simulink model "FSAC2021_V1_Running"  (R2014a)
settings: Solver=FixedStepDiscrete  StartTime=0.0  StopTime=inf  FixedStep=0.0005  RelTol=1e-3
model workspace (MAT data in the model file):
  MCOS : class17 (value not decoded)
  MCOS : class17 (value not decoded)
  MCOS : class17 (value not decoded)
  MCOS : class17 (value not decoded)
  MCOS : class17 (value not decoded)
  MCOS : class17 (value not decoded)
  MCOS : class17 (value not decoded)
  MCOS : class17 (value not decoded)
  MCOS : class17 (value not decoded)
  MCOS : class17 (value not decoded)
  MCOS : class17 (value not decoded)
  MCOS : class17 (value not decoded)
  MCOS : class17 (value not decoded)
  MCOS : class17 (value not decoded)
  MCOS : class17 (value not decoded)
  MCOS : class17 (value not decoded)
  MCOS : class17 (value not decoded)
  MCOS : class17 (value not decoded)
  MCOS : class17 (value not decoded)
  BUZZER_START = 1
  MCOS : class17 (value not decoded)
  MCOS : class17 (value not decoded)
  MCOS : class17 (value not decoded)
  MCOS : class17 (value not decoded)
  MCOS : class17 (value not decoded)
  MCOS : class17 (value not decoded)
  MCOS : class17 (value not decoded)
  MCOS : class17 (value not decoded)
  MCOS : class17 (value not decoded)
  MCOS : class17 (value not decoded)
  MCOS : class17 (value not decoded)
  MCOS : class17 (value not decoded)
  MCOS : class17 (value not decoded)
  MCOS : class17 (value not decoded)
  MCOS : class17 (value not decoded)
  MCOS : class17 (value not decoded)
  MCOS : class17 (value not decoded)
  MCOS : class17 (value not decoded)
  MCOS : class17 (value not decoded)
  MCOS : class17 (value not decoded)
  MCOS : class17 (value not decoded)
  MCOS : class17 (value not decoded)
  MCOS : class17 (value not decoded)
  MCOS : class17 (value not decoded)
  MCOS : class17 (value not decoded)
  MCOS : class17 (value not decoded)
  MCOS : class17 (value not decoded)
  MCOS : class17 (value not decoded)
  MCOS : class17 (value not decoded)
  MCOS : class17 (value not decoded)
  MCOS : class17 (value not decoded)
  MCOS : class17 (value not decoded)
  MCOS : class17 (value not decoded)
  MCOS : class17 (value not decoded)
  MCOS : class17 (value not decoded)
  MCOS : class17 (value not decoded)
  MCOS : class17 (value not decoded)
  MCOS : class17 (value not decoded)
  Brake = 11
  MCOS : class17 (value not decoded)
  MCOS : class17 (value not decoded)
  MCOS : class17 (value not decoded)
  MCOS : class17 (value not decoded)
  MCOS : class17 (value not decoded)
  MCOS : class17 (value not decoded)
  MCOS : class17 (value not decoded)
  MCOS : class17 (value not decoded)
  Sensor_Acc_b = 101.85
  Sensor_Acc_k = -0.0185
  Str_Sen_Orig_Angle = -341
  MCOS : class17 (value not decoded)
  Tire_D = 0.47
  T = 0.05
libraries: simulink x402, ec55xxlib x134
(part 3 of 17)

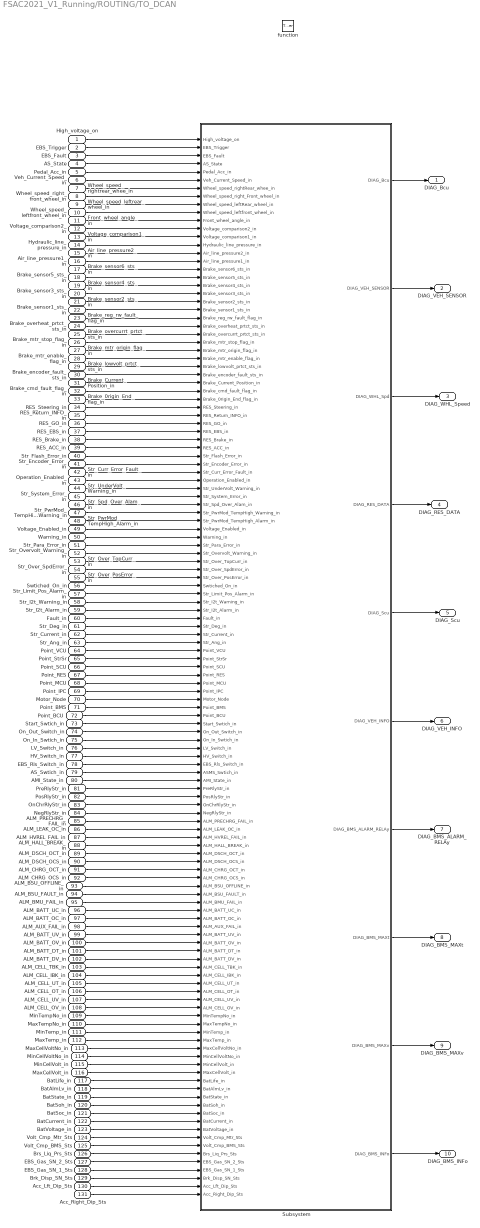
== system FSAC2021_V1_Running/ROUTING/TO_DCAN ==
  High_voltage_on : Inport
  EBS_Trigger : Inport  Port=2
  EBS_Fault : Inport  Port=3
  AS_State : Inport  Port=4
  Pedal_Acc_in : Inport  Port=5
  Veh_Current_Speed_in : Inport  Port=6
  Wheel_speed_rightrear_whee_in : Inport  Port=7
  Wheel_speed_right_front_wheel_in : Inport  Port=8
  Wheel_speed_leftrear_wheel_in : Inport  Port=9
  Wheel_speed_leftfront_wheel_in : Inport  Port=10
  Front_wheel_angle_in : Inport  Port=11
  Voltage_comparison2_in : Inport  Port=12
  Voltage_comparison1_in : Inport  Port=13
  Hydraulic_line_pressure_in : Inport  Port=14
  Air_line_pressure2_in : Inport  Port=15
  Air_line_pressure1_in : Inport  Port=16
  Brake_sensor6_sts_in : Inport  Port=17
  Brake_sensor5_sts_in : Inport  Port=18
  Brake_sensor4_sts_in : Inport  Port=19
  Brake_sensor3_sts_in : Inport  Port=20
  Brake_sensor2_sts_in : Inport  Port=21
  Brake_sensor1_sts_in : Inport  Port=22
  Brake_reg_rw_fault_flag_in : Inport  Port=23
  Brake_overheat_prtct_sts_in : Inport  Port=24
  Brake_overcurrt_prtct_sts_in : Inport  Port=25
  Brake_mtr_stop_flag_in : Inport  Port=26
  Brake_mtr_origin_flag_in : Inport  Port=27
  Brake_mtr_enable_flag_in : Inport  Port=28
  Brake_lowvolt_prtct_sts_in : Inport  Port=29
  Brake_encoder_fault_sts_in : Inport  Port=30
  Brake_Current_Position_in : Inport  Port=31
  Brake_cmd_fault_flag_in : Inport  Port=32
  Brake_0rigin_End_flag_in : Inport  Port=33
  RES_Steering_in : Inport  Port=34
  RES_Return_INFO_in : Inport  Port=35
  RES_GO_in : Inport  Port=36
  RES_EBS_in : Inport  Port=37
  RES_Brake_in : Inport  Port=38
  RES_ACC_in : Inport  Port=39
  Str_Flash_Error_in : Inport  Port=40
  Str_Encoder_Error_in : Inport  Port=41
  Str_Curr_Error_Fault_in : Inport  Port=42
  Operation_Enabled_in : Inport  Port=43
  Str_UnderVolt_Warning_in : Inport  Port=44
  Str_System_Error_in : Inport  Port=45
  Str_Spd_Over_Alam_in : Inport  Port=46
  Str_PwrMod_TempHigh_Warning_in : Inport  Port=47
  Str_PwrMod_TempHigh_Alarm_in : Inport  Port=48
  Voltage_Enabled_in : Inport  Port=49
  Warning_in : Inport  Port=50
  Str_Para_Error_in : Inport  Port=51
  Str_Overvolt_Warning_in : Inport  Port=52
  Str_Over_TopCurr_in : Inport  Port=53
  Str_Over_SpdError_in : Inport  Port=54
  Str_Over_PosError_in : Inport  Port=55
  Swtiched_On_in : Inport  Port=56
  Str_Limit_Pos_Alarm_in : Inport  Port=57
  Str_I2t_Warning_in : Inport  Port=58
  Str_I2t_Alarm_in : Inport  Port=59
  Fault_in : Inport  Port=60
  Str_Deg_in : Inport  Port=61
  Str_Current_in : Inport  Port=62
  Str_Ang_in : Inport  Port=63
  Point_VCU : Inport  Port=64
  Point_StrSr : Inport  Port=65
  Point_SCU : Inport  Port=66
  Point_RES : Inport  Port=67
  Point_MCU : Inport  Port=68
  Point_IPC : Inport  Port=69
  Motor_Node : Inport  Port=70
  Point_BMS : Inport  Port=71
  Point_BCU : Inport  Port=72
  Start_Swtich_in : Inport  Port=73
  On_Out_Switch_in : Inport  Port=74
  On_In_Swtich_in : Inport  Port=75
  LV_Switch_in : Inport  Port=76
  HV_Switch_in : Inport  Port=77
  EBS_Rls_Switch_in : Inport  Port=78
  AS_Swtich_in : Inport  Port=79
  AMI_State_in : Inport  Port=80
  PreRlyStr_in : Inport  Port=81
  PosRlyStr_in : Inport  Port=82
  OnChrRlyStr_in : Inport  Port=83
  NegRlyStr_in : Inport  Port=84
  ALM_PRECHRG_FAIL_in : Inport  Port=85
  ALM_LEAK_OC_in : Inport  Port=86
  ALM_HVREL_FAIL_in : Inport  Port=87
  ALM_HALL_BREAK_in : Inport  Port=88
  ALM_DSCH_OCT_in : Inport  Port=89
  ALM_DSCH_OCS_in : Inport  Port=90
  ALM_CHRG_OCT_in : Inport  Port=91
  ALM_CHRG_OCS_in : Inport  Port=92
  ALM_BSU_OFFLINE_in : Inport  Port=93
  ALM_BSU_FAULT_in : Inport  Port=94
  ALM_BMU_FAIL_in : Inport  Port=95
  ALM_BATT_UC_in : Inport  Port=96
  ALM_BATT_OC_in : Inport  Port=97
  ALM_AUX_FAIL_in : Inport  Port=98
  ALM_BATT_UV_in : Inport  Port=99
  ALM_BATT_OV_in : Inport  Port=100
  ALM_BATT_DT_in : Inport  Port=101
  ALM_BATT_DV_in : Inport  Port=102
  ALM_CELL_TBK_in : Inport  Port=103
  ALM_CELL_IBK_in : Inport  Port=104
  ALM_CELL_UT_in : Inport  Port=105
  ALM_CELL_OT_in : Inport  Port=106
  ALM_CELL_UV_in : Inport  Port=107
  ALM_CELL_OV_in : Inport  Port=108
  MinTempNo_in : Inport  Port=109
  MaxTempNo_in : Inport  Port=110
  MinTemp_in : Inport  Port=111
  MaxTemp_in : Inport  Port=112
  MaxCellVoltNo_in : Inport  Port=113
  MinCellVoltNo_in : Inport  Port=114
  MinCellVolt_in : Inport  Port=115
  MaxCellVolt_in : Inport  Port=116
  BatLife_in : Inport  Port=117
  BatAlmLv_in : Inport  Port=118
  BatState_in : Inport  Port=119
  BatSoh_in : Inport  Port=120
  BatSoc_in : Inport  Port=121
  BatCurrent_in : Inport  Port=122
  BatVoltage_in : Inport  Port=123
  Volt_Cmp_Mtr_Sts : Inport  Port=124
  Volt_Cmp_BMS_Sts : Inport  Port=125
  "Brs_Liq_Prs_Sts " : Inport  Port=126
  EBS_Gas_SN_2_Sts : Inport  Port=127
  EBS_Gas_SN_1_Sts : Inport  Port=128
  Brk_Disp_SN_Sts : Inport  Port=129
  Acc_Lft_Dip_Sts : Inport  Port=130
  Acc_Right_Dip_Sts : Inport  Port=131
  function : TriggerPort  TriggerType=function-call
  Subsystem : Subsystem
  DIAG_Bcu : Outport
  DIAG_VEH_SENSOR : Outport  Port=2
  DIAG_WHL_Speed : Outport  Port=3
  DIAG_RES_DATA : Outport  Port=4
  DIAG_Scu : Outport  Port=5
  DIAG_VEH_INFO : Outport  Port=6
  DIAG_BMS_ALARM_RELAy : Outport  Port=7
  DIAG_BMS_MAXt : Outport  Port=8
  DIAG_BMS_MAXv : Outport  Port=9
  DIAG_BMS_INFo : Outport  Port=10
  wires:
  High_voltage_on/1 -> Subsystem/1(High_voltage_on)
  EBS_Trigger/1 -> Subsystem/2(EBS_Trigger)
  EBS_Fault/1 -> Subsystem/3(EBS_Fault)
  AS_State/1 -> Subsystem/4(AS_State)
  Pedal_Acc_in/1 -> Subsystem/5(Pedal_Acc_in)
  Veh_Current_Speed_in/1 -> Subsystem/6(Veh_Current_Speed_in)
  Wheel_speed_rightrear_whee_in/1 -> Subsystem/7(Wheel_speed_rightRear_whee_in)
  Wheel_speed_right_front_wheel_in/1 -> Subsystem/8(Wheel_speed_right_Front_wheel_in)
  Wheel_speed_leftrear_wheel_in/1 -> Subsystem/9(Wheel_speed_leftRear_wheel_in)
  Wheel_speed_leftfront_wheel_in/1 -> Subsystem/10(Wheel_speed_leftfront_wheel_in)
  Front_wheel_angle_in/1 -> Subsystem/11(Front_wheel_angle_in)
  Voltage_comparison2_in/1 -> Subsystem/12(Voltage_comparison2_in)
  Voltage_comparison1_in/1 -> Subsystem/13(Voltage_comparison1_in)
  Hydraulic_line_pressure_in/1 -> Subsystem/14(Hydraulic_line_pressure_in)
  Air_line_pressure2_in/1 -> Subsystem/15(Air_line_pressure2_in)
  Air_line_pressure1_in/1 -> Subsystem/16(Air_line_pressure1_in)
  Brake_sensor6_sts_in/1 -> Subsystem/17(Brake_sensor6_sts_in)
  Brake_sensor5_sts_in/1 -> Subsystem/18(Brake_sensor5_sts_in)
  Brake_sensor4_sts_in/1 -> Subsystem/19(Brake_sensor4_sts_in)
  Brake_sensor3_sts_in/1 -> Subsystem/20(Brake_sensor3_sts_in)
  Brake_sensor2_sts_in/1 -> Subsystem/21(Brake_sensor2_sts_in)
  Brake_sensor1_sts_in/1 -> Subsystem/22(Brake_sensor1_sts_in)
  Brake_reg_rw_fault_flag_in/1 -> Subsystem/23(Brake_reg_rw_fault_flag_in)
  Brake_overheat_prtct_sts_in/1 -> Subsystem/24(Brake_overheat_prtct_sts_in)
  Brake_overcurrt_prtct_sts_in/1 -> Subsystem/25(Brake_overcurrt_prtct_sts_in)
  Brake_mtr_stop_flag_in/1 -> Subsystem/26(Brake_mtr_stop_flag_in)
  Brake_mtr_origin_flag_in/1 -> Subsystem/27(Brake_mtr_origin_flag_in)
  Brake_mtr_enable_flag_in/1 -> Subsystem/28(Brake_mtr_enable_flag_in)
  Brake_lowvolt_prtct_sts_in/1 -> Subsystem/29(Brake_lowvolt_prtct_sts_in)
  Brake_encoder_fault_sts_in/1 -> Subsystem/30(Brake_encoder_fault_sts_in)
  Brake_Current_Position_in/1 -> Subsystem/31(Brake_Current_Position_in)
  Brake_cmd_fault_flag_in/1 -> Subsystem/32(Brake_cmd_fault_flag_in)
  Brake_0rigin_End_flag_in/1 -> Subsystem/33(Brake_0rigin_End_flag_in)
  RES_Steering_in/1 -> Subsystem/34(RES_Steering_in)
  RES_Return_INFO_in/1 -> Subsystem/35(RES_Return_INFO_in)
  RES_GO_in/1 -> Subsystem/36(RES_GO_in)
  RES_EBS_in/1 -> Subsystem/37(RES_EBS_in)
  RES_Brake_in/1 -> Subsystem/38(RES_Brake_in)
  RES_ACC_in/1 -> Subsystem/39(RES_ACC_in)
  Str_Flash_Error_in/1 -> Subsystem/40(Str_Flash_Error_in)
  Str_Encoder_Error_in/1 -> Subsystem/41(Str_Encoder_Error_in)
  Str_Curr_Error_Fault_in/1 -> Subsystem/42(Str_Curr_Error_Fault_in)
  Operation_Enabled_in/1 -> Subsystem/43(Operation_Enabled_in)
  Str_UnderVolt_Warning_in/1 -> Subsystem/44(Str_UnderVolt_Warning_in)
  Str_System_Error_in/1 -> Subsystem/45(Str_System_Error_in)
  Str_Spd_Over_Alam_in/1 -> Subsystem/46(Str_Spd_Over_Alam_in)
  Str_PwrMod_TempHigh_Warning_in/1 -> Subsystem/47(Str_PwrMod_TempHigh_Warning_in)
  Str_PwrMod_TempHigh_Alarm_in/1 -> Subsystem/48(Str_PwrMod_TempHigh_Alarm_in)
  Voltage_Enabled_in/1 -> Subsystem/49(Voltage_Enabled_in)
  Warning_in/1 -> Subsystem/50(Warning_in)
  Str_Para_Error_in/1 -> Subsystem/51(Str_Para_Error_in)
  Str_Overvolt_Warning_in/1 -> Subsystem/52(Str_Overvolt_Warning_in)
  Str_Over_TopCurr_in/1 -> Subsystem/53(Str_Over_TopCurr_in)
  Str_Over_SpdError_in/1 -> Subsystem/54(Str_Over_SpdError_in)
  Str_Over_PosError_in/1 -> Subsystem/55(Str_Over_PosError_in)
  Swtiched_On_in/1 -> Subsystem/56(Swtiched_On_in)
  Str_Limit_Pos_Alarm_in/1 -> Subsystem/57(Str_Limit_Pos_Alarm_in)
  Str_I2t_Warning_in/1 -> Subsystem/58(Str_I2t_Warning_in)
  Str_I2t_Alarm_in/1 -> Subsystem/59(Str_I2t_Alarm_in)
  Fault_in/1 -> Subsystem/60(Fault_in)
  Str_Deg_in/1 -> Subsystem/61(Str_Deg_in)
  Str_Current_in/1 -> Subsystem/62(Str_Current_in)
  Str_Ang_in/1 -> Subsystem/63(Str_Ang_in)
  Point_VCU/1 -> Subsystem/64(Point_VCU)
  Point_StrSr/1 -> Subsystem/65(Point_StrSr)
  Point_SCU/1 -> Subsystem/66(Point_SCU)
  Point_RES/1 -> Subsystem/67(Point_RES)
  Point_MCU/1 -> Subsystem/68(Point_MCU)
  Point_IPC/1 -> Subsystem/69(Point_IPC)
  Point_BMS/1 -> Subsystem/71(Point_BMS)
  Point_BCU/1 -> Subsystem/72(Point_BCU)
  Start_Swtich_in/1 -> Subsystem/73(Start_Swtich_in)
  On_Out_Switch_in/1 -> Subsystem/74(On_Out_Switch_in)
  On_In_Swtich_in/1 -> Subsystem/75(On_In_Swtich_in)
  LV_Switch_in/1 -> Subsystem/76(LV_Switch_in)
  HV_Switch_in/1 -> Subsystem/77(HV_Switch_in)
  EBS_Rls_Switch_in/1 -> Subsystem/78(EBS_Rls_Switch_in)
  AS_Swtich_in/1 -> Subsystem/79(ASMS_Swtich_in)
  AMI_State_in/1 -> Subsystem/80(AMI_State_in)
  PreRlyStr_in/1 -> Subsystem/81(PreRlyStr_in)
  PosRlyStr_in/1 -> Subsystem/82(PosRlyStr_in)
  OnChrRlyStr_in/1 -> Subsystem/83(OnChrRlyStr_in)
  NegRlyStr_in/1 -> Subsystem/84(NegRlyStr_in)
  ALM_PRECHRG_FAIL_in/1 -> Subsystem/85(ALM_PRECHRG_FAIL_in)
  ALM_LEAK_OC_in/1 -> Subsystem/86(ALM_LEAK_OC_in)
  ALM_HVREL_FAIL_in/1 -> Subsystem/87(ALM_HVREL_FAIL_in)
  ALM_HALL_BREAK_in/1 -> Subsystem/88(ALM_HALL_BREAK_in)
  ALM_DSCH_OCT_in/1 -> Subsystem/89(ALM_DSCH_OCT_in)
  ALM_DSCH_OCS_in/1 -> Subsystem/90(ALM_DSCH_OCS_in)
  ALM_CHRG_OCT_in/1 -> Subsystem/91(ALM_CHRG_OCT_in)
  ALM_CHRG_OCS_in/1 -> Subsystem/92(ALM_CHRG_OCS_in)
  ALM_BSU_OFFLINE_in/1 -> Subsystem/93(ALM_BSU_OFFLINE_in)
  ALM_BSU_FAULT_in/1 -> Subsystem/94(ALM_BSU_FAULT_in)
  ALM_BMU_FAIL_in/1 -> Subsystem/95(ALM_BMU_FAIL_in)
  ALM_BATT_UC_in/1 -> Subsystem/96(ALM_BATT_UC_in)
  ALM_BATT_OC_in/1 -> Subsystem/97(ALM_BATT_OC_in)
  ALM_AUX_FAIL_in/1 -> Subsystem/98(ALM_AUX_FAIL_in)
  ALM_BATT_UV_in/1 -> Subsystem/99(ALM_BATT_UV_in)
  ALM_BATT_OV_in/1 -> Subsystem/100(ALM_BATT_OV_in)
  ALM_BATT_DT_in/1 -> Subsystem/101(ALM_BATT_DT_in)
  ALM_BATT_DV_in/1 -> Subsystem/102(ALM_BATT_DV_in)
  ALM_CELL_TBK_in/1 -> Subsystem/103(ALM_CELL_TBK_in)
  ALM_CELL_IBK_in/1 -> Subsystem/104(ALM_CELL_IBK_in)
  ALM_CELL_UT_in/1 -> Subsystem/105(ALM_CELL_UT_in)
  ALM_CELL_OT_in/1 -> Subsystem/106(ALM_CELL_OT_in)
  ALM_CELL_UV_in/1 -> Subsystem/107(ALM_CELL_UV_in)
  ALM_CELL_OV_in/1 -> Subsystem/108(ALM_CELL_OV_in)
  MinTempNo_in/1 -> Subsystem/109(MinTempNo_in)
  MaxTempNo_in/1 -> Subsystem/110(MaxTempNo_in)
  MinTemp_in/1 -> Subsystem/111(MinTemp_in)
  MaxTemp_in/1 -> Subsystem/112(MaxTemp_in)
  MaxCellVoltNo_in/1 -> Subsystem/113(MaxCellVoltNo_in)
  MinCellVoltNo_in/1 -> Subsystem/114(MinCellVoltNo_in)
  MinCellVolt_in/1 -> Subsystem/115(MinCellVolt_in)
  MaxCellVolt_in/1 -> Subsystem/116(MaxCellVolt_in)
  BatLife_in/1 -> Subsystem/117(BatLife_in)
  BatAlmLv_in/1 -> Subsystem/118(BatAlmLv_in)
  BatState_in/1 -> Subsystem/119(BatState_in)
  BatSoh_in/1 -> Subsystem/120(BatSoh_in)
  BatSoc_in/1 -> Subsystem/121(BatSoc_in)
  BatCurrent_in/1 -> Subsystem/122(BatCurrent_in)
  BatVoltage_in/1 -> Subsystem/123(BatVoltage_in)
  Subsystem/1(DIAG_Bcu) -> DIAG_Bcu/1
  Subsystem/2("DIAG_VEH_SENSOR ") -> DIAG_VEH_SENSOR/1
  Subsystem/3(DIAG_WHL_Spd) -> DIAG_WHL_Speed/1
  Subsystem/4(DIAG_RES_DATA) -> DIAG_RES_DATA/1
  Subsystem/5(DIAG_Scu) -> DIAG_Scu/1
  Subsystem/6("DIAG_VEH_INFO ") -> DIAG_VEH_INFO/1
  Subsystem/7(DIAG_BMS_ALARM_RELAy) -> DIAG_BMS_ALARM_RELAy/1
  Subsystem/8(DIAG_BMS_MAXt) -> DIAG_BMS_MAXt/1
  Subsystem/9(DIAG_BMS_MAXv) -> DIAG_BMS_MAXv/1
  Subsystem/10(DIAG_BMS_INFo) -> DIAG_BMS_INFo/1
  Motor_Node/1 -> Subsystem/70(Motor_Node)
  Volt_Cmp_Mtr_Sts/1 -> Subsystem/124(Volt_Cmp_Mtr_Sts)
  Volt_Cmp_BMS_Sts/1 -> Subsystem/125(Volt_Cmp_BMS_Sts)
  "Brs_Liq_Prs_Sts "/1 -> Subsystem/126("Brs_Liq_Prs_Sts ")
  EBS_Gas_SN_2_Sts/1 -> Subsystem/127(EBS_Gas_SN_2_Sts)
  EBS_Gas_SN_1_Sts/1 -> Subsystem/128(EBS_Gas_SN_1_Sts)
  Brk_Disp_SN_Sts/1 -> Subsystem/129(Brk_Disp_SN_Sts)
  Acc_Lft_Dip_Sts/1 -> Subsystem/130(Acc_Lft_Dip_Sts)
  Acc_Right_Dip_Sts/1 -> Subsystem/131(Acc_Right_Dip_Sts)

== system FSAC2021_V1_Running/ROUTING/TO_PCAN ==
  function : TriggerPort  TriggerType=function-call

== system FSAC2021_V1_Running/VCU_CAN_Read/DCAN_REC ==
  DIAG_VCU_CTRL : ec55xxlib/RapidECU_U2/07CANCommucation/CANReceive  canmodule=C  canbuffer=54  canmessageid=1937  canmessagetype=Standard(11-bit ID)  datalength=4  sampletime=Ts
  DIAG_VCU_CTRL1 : Subsystem
  Terminator4 : Terminator
  Terminator5 : Terminator
  tag scope: DCAN_Ctr_Flag=global, DCAN_Data_Flag=global, TEST_Acc=global, TEST_Brake=global, TEST_EBS=global, TEST_Go=global, TEST_Steer=global
  wires:
  DIAG_VCU_CTRL/4 -> DIAG_VCU_CTRL1/1(input)
  DIAG_VCU_CTRL/2 -> [DCAN_Data_Flag]
  DIAG_VCU_CTRL/3 -> Terminator4/1
  DIAG_VCU_CTRL/5 -> Terminator5/1
  DIAG_VCU_CTRL1/3(TEST_Go_Out) -> [TEST_Go]
  DIAG_VCU_CTRL1/4(TEST_EBS_Out) -> [TEST_EBS]
  DIAG_VCU_CTRL1/2(TEST_Steer_Out) -> [TEST_Steer]
  DIAG_VCU_CTRL1/5(TEST_Brake_Out) -> [TEST_Brake]
  DIAG_VCU_CTRL1/6(TEST_Acc_Out) -> [TEST_Acc]
  DIAG_VCU_CTRL/1 -> DIAG_VCU_CTRL1/Trigger
  DIAG_VCU_CTRL1/1(Vel_Ctrl_Req_Out) -> [DCAN_Ctr_Flag]

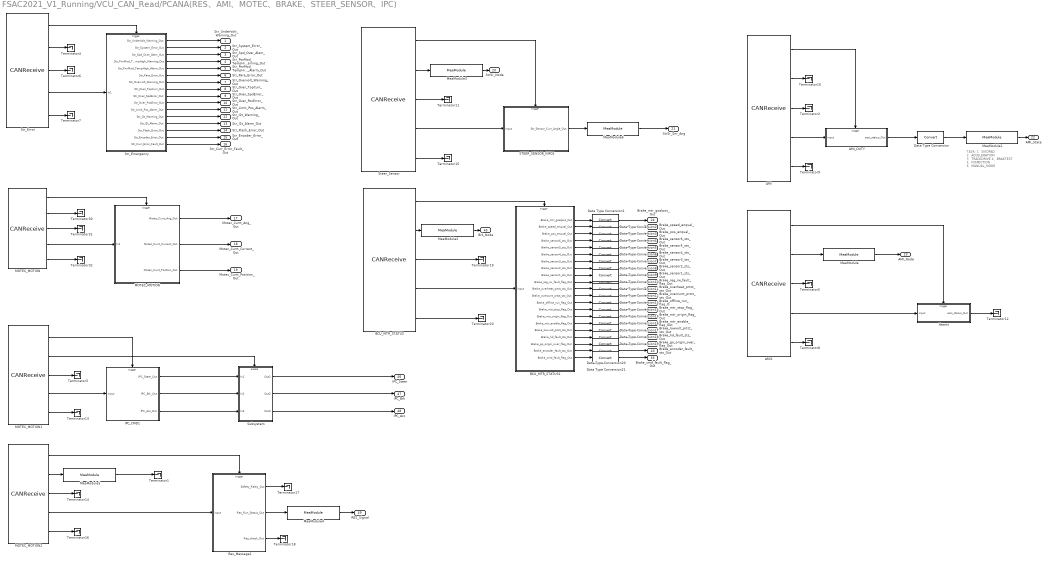
== system FSAC2021_V1_Running/VCU_CAN_Read/PCANA(RES、AMI、MOTEC、BRAKE、STEER_SENSOR、IPC) ==
  note: TASK:
      | 1、SKIDPAD
      | 2、ACCELERATION
      | 3、TRACKDRIVE
      | 4、BRAKTEST
      | 5、INSPECTION
      | 6、MANUAL_MODE
  AMI : ec55xxlib/RapidECU_U2/07CANCommucation/CANReceive  canmodule=A  canbuffer=16  canmessageid=1169  canmessagetype=Standard(11-bit ID)  datalength=1  sampletime=0.05
  AMI1 : ec55xxlib/RapidECU_U2/07CANCommucation/CANReceive  canmodule=A  canbuffer=26  canmessageid=1168  canmessagetype=Standard(11-bit ID)  datalength=1  sampletime=0.05
  AMI_DUTY : Subsystem
  BCU_MTR_STATUS : ec55xxlib/RapidECU_U2/07CANCommucation/CANReceive  canmodule=A  canbuffer=21  canmessageid=257  canmessagetype=Standard(11-bit ID)  datalength=8  sampletime=0.01
  BCU_MTR_STATUS1 : Subsystem
  Data Type Conversion{,1..21} (22 alike) : DataTypeConversion
  Heartt : Subsystem
  IPC_CMD1 : Subsystem
  MOTEC_MOTION : ec55xxlib/RapidECU_U2/07CANCommucation/CANReceive  canmodule=A  canbuffer=5  canmessageid=641  canmessagetype=Standard(11-bit ID)  datalength=8  sampletime=0.5
  "MOTEC_MOTION " : Subsystem
  MOTEC_MOTION1 : ec55xxlib/RapidECU_U2/07CANCommucation/CANReceive  canmodule=A  canbuffer=41  canmessageid=256  canmessagetype=Standard(11-bit ID)  datalength=3  sampletime=0.01
  MOTEC_MOTION2 : ec55xxlib/RapidECU_U2/07CANCommucation/CANReceive  canmodule=A  canbuffer=35  canmessageid=279  canmessagetype=Standard(11-bit ID)  datalength=1  sampletime=0.01
  MeaModule : ec55xxlib/RapidECU_U2/11Calibration/MeaModule  signal=AMI_HEART
  MeaModule1 : ec55xxlib/RapidECU_U2/11Calibration/MeaModule  signal=AMI
  MeaModule2 : ec55xxlib/RapidECU_U2/11Calibration/MeaModule  signal=brake_node
  MeaModule3 : ec55xxlib/RapidECU_U2/11Calibration/MeaModule  signal=strsr_node
  MeaModule4 : ec55xxlib/RapidECU_U2/11Calibration/MeaModule  signal=RES_Value
  MeaModule5 : ec55xxlib/RapidECU_U2/11Calibration/MeaModule  signal=RES__ok
  MeaModule6 : ec55xxlib/RapidECU_U2/11Calibration/MeaModule  signal=Steer_sensor_angle
  Res_Message1 : Subsystem
  STEER_SENSOR_INFO1 : Subsystem
  Steer_Sensor : ec55xxlib/RapidECU_U2/07CANCommucation/CANReceive  canmodule=A  canbuffer=38  canmessageid=485  canmessagetype=Standard(11-bit ID)  datalength=8  sampletime=0.01
  "Str_Emergency " : Subsystem
  Str_Error : ec55xxlib/RapidECU_U2/07CANCommucation/CANReceive  canmodule=A  canbuffer=4  canmessageid=129  canmessagetype=Standard(11-bit ID)  datalength=8  sampletime=-1
  Subsystem : Subsystem
  Terminator{1..20,30..32} (23 alike) : Terminator
  Str_UnderVolt_Warning_Out : Outport
  Str_System_Error_Out : Outport  Port=2
  Str_Spd_Over_Alam_Out : Outport  Port=3
  Str_PwrMod_TempHigh_Warning_Out : Outport  Port=4
  Str_PwrMod_TempHigh_Alarm_Out : Outport  Port=5
  Str_Para_Error_Out : Outport  Port=6
  Str_Overvolt_Warning_Out : Outport  Port=7
  Str_Over_TopCurr_Out : Outport  Port=8
  Str_Over_SpdError_Out : Outport  Port=9
  Str_Over_PosError_Out : Outport  Port=10
  Str_Limit_Pos_Alarm_Out : Outport  Port=11
  Str_I2t_Warning_Out : Outport  Port=12
  Str_I2t_Alarm_Out : Outport  Port=13
  Str_Flash_Error_Out : Outport  Port=14
  Str_Encoder_Error_Out : Outport  Port=15
  Str_Curr_Error_Fault_Out : Outport  Port=16
  Motec_Currt_Ang_Out : Outport  Port=17
  Motec_Currt_Current_Out : Outport  Port=18
  Motec_Currt_Position_Out : Outport  Port=19
  StrSr_Node : Outport  Port=20
  StrSr_Snr_Ang : Outport  Port=21
  AMI_State : Outport  Port=22
  AMI_Node : Outport  Port=23
  Brake_mtr_goalpos_Out : Outport  Port=24
  Brake_speed_enqual_Out : Outport  Port=25
  Brake_pos_enqual_Out : Outport  Port=26
  Brake_sensor6_sts_Out : Outport  Port=27
  Brake_sensor5_sts_Out : Outport  Port=28
  Brake_sensor4_sts_Out : Outport  Port=29
  Brake_sensor3_sts_Out : Outport  Port=30
  Brake_sensor2_sts_Out : Outport  Port=31
  Brake_sensor1_sts_Out : Outport  Port=32
  Brake_reg_rw_fault_flag_Out : Outport  Port=33
  Brake_overheat_prtct_sts_Out : Outport  Port=34
  Brake_overcurrt_prtct_sts_Out : Outport  Port=35
  Brake_offline_run_flag_O : Outport  Port=36
  Brake_mtr_stop_flag_Out : Outport  Port=37
  Brake_mtr_origin_flag_Out : Outport  Port=38
  Brake_mtr_enable_flag_Out : Outport  Port=39
  Brake_lowvolt_prtct_sts_Out : Outport  Port=40
  Brake_hd_fault_sts_Out : Outport  Port=41
  Brake_go_origin_over_flag_Out : Outport  Port=42
  Brake_encoder_fault_sts_Out : Outport  Port=43
  Brake_cmd_fault_flag_Out : Outport  Port=44
  Brk_Node : Outport  Port=45
  IPC_Steer : Outport  Port=46
  IPC_Brk : Outport  Port=47
  IPC_Acc : Outport  Port=48
  RES_Signal : Outport  Port=49
  wires:
  Steer_Sensor/1 -> STEER_SENSOR_INFO1/Trigger
  Steer_Sensor/4 -> STEER_SENSOR_INFO1/1(input)
  Steer_Sensor/2 -> MeaModule3/1
  STEER_SENSOR_INFO1/1(Str_Sensor_Curr_Angle_Out) -> MeaModule6/1
  Steer_Sensor/3 -> Terminator11/1
  Steer_Sensor/5 -> Terminator15/1
  AMI/2 -> Terminator10/1
  AMI/5 -> Terminator9/1
  AMI/1 -> AMI_DUTY/Trigger
  AMI_DUTY/1(assi_status_Out) -> Data Type Conversion/1
  Data Type Conversion/1 -> MeaModule1/1
  AMI/4 -> AMI_DUTY/1(input)
  AMI/3 -> Terminator2/1
  AMI1/4 -> Heartt/1(input)
  AMI1/3 -> Terminator5/1
  AMI1/5 -> Terminator8/1
  AMI1/1 -> Heartt/Trigger
  AMI1/2 -> MeaModule/1
  Heartt/1(assi_status_Out) -> Terminator12/1
  "Str_Emergency "/3(Str_Spd_Over_Alam_Out) -> Str_Spd_Over_Alam_Out/1
  "Str_Emergency "/15(Str_Encoder_Error_Out) -> Str_Encoder_Error_Out/1
  "Str_Emergency "/2(Str_System_Error_Out) -> Str_System_Error_Out/1
  "Str_Emergency "/13(Str_I2t_Alarm_Out) -> Str_I2t_Alarm_Out/1
  "Str_Emergency "/6(Str_Para_Error_Out) -> Str_Para_Error_Out/1
  "Str_Emergency "/5(Str_PwrMod_TempHigh_Alarm_Out) -> Str_PwrMod_TempHigh_Alarm_Out/1
  "Str_Emergency "/12(Str_I2t_Warning_Out) -> Str_I2t_Warning_Out/1
  Str_Error/5 -> Terminator7/1
  "Str_Emergency "/10(Str_Over_PosError_Out) -> Str_Over_PosError_Out/1
  Str_Error/4 -> "Str_Emergency "/1(In1)
  Str_Error/2 -> Terminator4/1
  "Str_Emergency "/7(Str_Overvolt_Warning_Out) -> Str_Overvolt_Warning_Out/1
  "Str_Emergency "/1(Str_UnderVolt_Warning_Out) -> Str_UnderVolt_Warning_Out/1
  "Str_Emergency "/11(Str_Limit_Pos_Alarm_Out) -> Str_Limit_Pos_Alarm_Out/1
  "Str_Emergency "/9(Str_Over_SpdError_Out) -> Str_Over_SpdError_Out/1
  Str_Error/3 -> Terminator6/1
  "Str_Emergency "/4(Str_PwrMod_TempHigh_Warning_Out) -> Str_PwrMod_TempHigh_Warning_Out/1
  "Str_Emergency "/16(Str_Curr_Error_Fault_Out) -> Str_Curr_Error_Fault_Out/1
  "Str_Emergency "/8(Str_Over_TopCurr_Out) -> Str_Over_TopCurr_Out/1
  "Str_Emergency "/14(Str_Flash_Error_Out) -> Str_Flash_Error_Out/1
  Str_Error/1 -> "Str_Emergency "/Trigger
  MOTEC_MOTION/5 -> Terminator32/1
  "MOTEC_MOTION "/1(Motec_Currt_Ang_Out) -> Motec_Currt_Ang_Out/1
  "MOTEC_MOTION "/3(Motec_Currt_Position_Out) -> Motec_Currt_Position_Out/1
  MOTEC_MOTION/4 -> "MOTEC_MOTION "/1(In1)
  MOTEC_MOTION/3 -> Terminator31/1
  MOTEC_MOTION/2 -> Terminator30/1
  "MOTEC_MOTION "/2(Motec_Currt_Current_Out) -> Motec_Currt_Current_Out/1
  MOTEC_MOTION/1 -> "MOTEC_MOTION "/Trigger
  MeaModule3/1 -> StrSr_Node/1
  MeaModule6/1 -> StrSr_Snr_Ang/1
  MeaModule1/1 -> AMI_State/1
  MeaModule/1 -> AMI_Node/1
  BCU_MTR_STATUS1/13(Brake_offline_run_flag_Out) -> Data Type Conversion13/1
  BCU_MTR_STATUS1/2(Brake_speed_enqual_Out) -> Data Type Conversion2/1
  BCU_MTR_STATUS/5 -> Terminator20/1
  BCU_MTR_STATUS1/16(Brake_mtr_enable_flag_Out) -> Data Type Conversion16/1
  BCU_MTR_STATUS/3 -> Terminator19/1
  BCU_MTR_STATUS/2 -> MeaModule2/1
  BCU_MTR_STATUS1/5(Brake_sensor5_sts_Out) -> Data Type Conversion5/1
  BCU_MTR_STATUS1/14(Brake_mtr_stop_flag_Out) -> Data Type Conversion14/1
  BCU_MTR_STATUS1/17(Brake_lowvolt_prtct_sts_Out) -> Data Type Conversion17/1
  BCU_MTR_STATUS/4 -> BCU_MTR_STATUS1/1(input)
  BCU_MTR_STATUS1/1(Brake_mtr_goalpos_Out) -> Data Type Conversion1/1
  BCU_MTR_STATUS1/18(Brake_hd_fault_sts_Out) -> Data Type Conversion18/1
  BCU_MTR_STATUS1/12(Brake_overcurrt_prtct_sts_Out) -> Data Type Conversion12/1
  BCU_MTR_STATUS1/19(Brake_go_origin_over_flag_Out) -> Data Type Conversion19/1
  BCU_MTR_STATUS/1 -> BCU_MTR_STATUS1/Trigger
  BCU_MTR_STATUS1/6(Brake_sensor4_sts_Out) -> Data Type Conversion6/1
  BCU_MTR_STATUS1/4(Brake_sensor6_sts_Out) -> Data Type Conversion4/1
  BCU_MTR_STATUS1/8(Brake_sensor2_sts_Out) -> Data Type Conversion8/1
  BCU_MTR_STATUS1/3(Brake_pos_enqual_Out) -> Data Type Conversion3/1
  BCU_MTR_STATUS1/10(Brake_reg_rw_fault_flag_Out) -> Data Type Conversion10/1
  BCU_MTR_STATUS1/20(Brake_encoder_fault_sts_Out) -> Data Type Conversion20/1
  BCU_MTR_STATUS1/21(Brake_cmd_fault_flag_Out) -> Data Type Conversion21/1
  BCU_MTR_STATUS1/9(Brake_sensor1_sts_Out) -> Data Type Conversion9/1
  BCU_MTR_STATUS1/15(Brake_mtr_origin_flag_Out) -> Data Type Conversion15/1
  BCU_MTR_STATUS1/11(Brake_overheat_prtct_sts_Out) -> Data Type Conversion11/1
  BCU_MTR_STATUS1/7(Brake_sensor3_sts_Out) -> Data Type Conversion7/1
  Data Type Conversion17/1 -> Brake_lowvolt_prtct_sts_Out/1
  Data Type Conversion1/1 -> Brake_mtr_goalpos_Out/1
  Data Type Conversion11/1 -> Brake_overheat_prtct_sts_Out/1
  Data Type Conversion13/1 -> Brake_offline_run_flag_O/1
  Data Type Conversion12/1 -> Brake_overcurrt_prtct_sts_Out/1
  Data Type Conversion10/1 -> Brake_reg_rw_fault_flag_Out/1
  Data Type Conversion16/1 -> Brake_mtr_enable_flag_Out/1
  Data Type Conversion14/1 -> Brake_mtr_stop_flag_Out/1
  Data Type Conversion18/1 -> Brake_hd_fault_sts_Out/1
  Data Type Conversion4/1 -> Brake_sensor6_sts_Out/1
  Data Type Conversion5/1 -> Brake_sensor5_sts_Out/1
  Data Type Conversion6/1 -> Brake_sensor4_sts_Out/1
  Data Type Conversion7/1 -> Brake_sensor3_sts_Out/1
  Data Type Conversion15/1 -> Brake_mtr_origin_flag_Out/1
  Data Type Conversion2/1 -> Brake_speed_enqual_Out/1
  Data Type Conversion8/1 -> Brake_sensor2_sts_Out/1
  Data Type Conversion19/1 -> Brake_go_origin_over_flag_Out/1
  Data Type Conversion9/1 -> Brake_sensor1_sts_Out/1
  Data Type Conversion21/1 -> Brake_cmd_fault_flag_Out/1
  Data Type Conversion3/1 -> Brake_pos_enqual_Out/1
  Data Type Conversion20/1 -> Brake_encoder_fault_sts_Out/1
  MeaModule2/1 -> Brk_Node/1
  MOTEC_MOTION1/4 -> IPC_CMD1/1(input)
  MOTEC_MOTION1/1 -> IPC_CMD1/Trigger
  MOTEC_MOTION1/3 -> Terminator3/1
  MOTEC_MOTION1/5 -> Terminator13/1
  Subsystem/3(Out3) -> IPC_Acc/1
  Subsystem/2(Out2) -> IPC_Brk/1
  IPC_CMD1/1(IPC_Steer_Out) -> Subsystem/1(In1)
  IPC_CMD1/2(IPC_Brk_Out) -> Subsystem/2(In2)
  IPC_CMD1/3(IPC_Acc_Out) -> Subsystem/3(In3)
  MOTEC_MOTION1/2 -> Subsystem/Enable
  Subsystem/1(Out1) -> IPC_Steer/1
  MOTEC_MOTION2/1 -> Res_Message1/Trigger
  MOTEC_MOTION2/2 -> MeaModule5/1
  MOTEC_MOTION2/3 -> Terminator14/1
  MOTEC_MOTION2/4 -> Res_Message1/1(input)
  MOTEC_MOTION2/5 -> Terminator16/1
  Res_Message1/1(Safety_Relay_Out) -> Terminator17/1
  Res_Message1/3(Res_check_Out) -> Terminator18/1
  Res_Message1/2(Res_Run_Status_Out) -> MeaModule4/1
  MeaModule4/1 -> RES_Signal/1
  MeaModule5/1 -> Terminator1/1

== system FSAC2021_V1_Running/VCU_CAN_Read/PCANB(BMS、DRIVE_MOTOR) ==
  function : TriggerPort  TriggerType=function-call
  BMS_ALARM : ec55xxlib/RapidECU_U2/07CANCommucation/CANReceive  canmodule=B  canbuffer=50  canmessageid=2556772595  canmessagetype=Extended(29-bit ID)  datalength=8  sampletime=-1
  "BMS_ALARM " : Subsystem
  BMS_HCU_MAXT : ec55xxlib/RapidECU_U2/07CANCommucation/CANReceive  canmodule=B  canbuffer=18  canmessageid=2556575987  canmessagetype=Extended(29-bit ID)  datalength=8  sampletime=-1
  BMS_HCU_MAXT1 : Subsystem
  BMS_HCU_MAXV : ec55xxlib/RapidECU_U2/07CANCommucation/CANReceive  canmodule=B  canbuffer=16  canmessageid=2556510451  canmessagetype=Extended(29-bit ID)  datalength=8  sampletime=-1
  "BMS_HCU_MAXV " : Subsystem
  BMS_HCU_POWER : ec55xxlib/RapidECU_U2/07CANCommucation/CANReceive  canmodule=B  canbuffer=52  canmessageid=2556707059  canmessagetype=Extended(29-bit ID)  datalength=8  sampletime=-1
  "BMS_HCU_POWER " : Subsystem
  BMS_RELAY : ec55xxlib/RapidECU_U2/07CANCommucation/CANReceive  canmodule=B  canbuffer=51  canmessageid=2556641523  canmessagetype=Extended(29-bit ID)  datalength=8  sampletime=-1
  "BMS_RELAY " : Subsystem
  MOTOR_CURRENT_SPEED : Subsystem
  MeaModule : ec55xxlib/RapidECU_U2/11Calibration/MeaModule  signal=motor_node
  "Motor_Current_Speed " : ec55xxlib/RapidECU_U2/07CANCommucation/CANReceive  canmodule=B  canbuffer=21  canmessageid=2147553443  canmessagetype=Extended(29-bit ID)  datalength=2  sampletime=-1
  Terminator{2,8..10,12..14,21..22,24..29,42..43} (17 alike) : Terminator
  heatingctl : Outport
  coolingctl : Outport  Port=2
  mintempno : Outport  Port=3
  maxtempno : Outport  Port=4
  mintemp : Outport  Port=5
  maxtemp : Outport  Port=6
  maxcellvoltno : Outport  Port=7
  mincellvoltno : Outport  Port=8
  mincellvolt : Outport  Port=9
  maxcellvolt : Outport  Port=10
  offChrRlyStr_Out : Outport  Port=11
  ChrReqCurr_Out : Outport  Port=12
  ChrReqVolt_Out : Outport  Port=13
  chrONCC_Out : Outport  Port=14
  chrOFFCC2_Out : Outport  Port=15
  ChrCommunication_Out : Outport  Port=16
  ChrState_Out : Outport  Port=17
  OnChrRlyStr_Out : Outport  Port=18
  PreRlyStr_Out : Outport  Port=19
  NegRlyStr_Out : Outport  Port=20
  PosRlyStr_Out : Outport  Port=21
  MaxDisPowerLimit_Out : Outport  Port=22
  MaxChrPowerLimit_Out : Outport  Port=23
  MaxDisCurtLimit_Out : Outport  Port=24
  MaxChrCurtLimit_Out : Outport  Port=25
  Motor_Node : Outport  Port=26
  Motor_Current_Speed : Outport  Port=27
  ALM_VCU_OFFLINE_Out : Outport  Port=28
  ALM_PRECHRG_FAIL_Out : Outport  Port=29
  ALM_LEAK_OC_Out : Outport  Port=30
  ALM_HVREL_FAIL_Out : Outport  Port=31
  ALM_HALL_BREAK_Out : Outport  Port=32
  ALM_DSCH_OCT_Out : Outport  Port=33
  ALM_DSCH_OCS_Out : Outport  Port=34
  ALM_CHRG_OCT_Out : Outport  Port=35
  ALM_CHRG_OCS_Out : Outport  Port=36
  ALM_BSU_OFFLINE_Out : Outport  Port=37
  ALM_BSU_FAULT_Out : Outport  Port=38
  ALM_BMU_FAIL_Out : Outport  Port=39
  ALM_BATT_UC_Out : Outport  Port=40
  ALM_BATT_OC_Out : Outport  Port=41
  ALM_AUX_FAIL_Out : Outport  Port=42
  ALM_BATT_UV_Out : Outport  Port=43
  ALM_BATT_OV_Out : Outport  Port=44
  ALM_BATT_DT_Out : Outport  Port=45
  ALM_BATT_DV_Out : Outport  Port=46
  ALM_CELL_TBK_Out : Outport  Port=47
  ALM_CELL_IBK_Out : Outport  Port=48
  ALM_CELL_UT_Out : Outport  Port=49
  ALM_CELL_OT_Out : Outport  Port=50
  ALM_CELL_UV_Out : Outport  Port=51
  ALM_CELL_OV_Out : Outport  Port=52
  wires:
  BMS_ALARM/5 -> Terminator42/1
  BMS_ALARM/1 -> "BMS_ALARM "/Trigger
  BMS_ALARM/3 -> Terminator9/1
  BMS_ALARM/2 -> Terminator8/1
  BMS_ALARM/4 -> "BMS_ALARM "/1(In1)
  BMS_RELAY/1 -> "BMS_RELAY "/Trigger
  BMS_RELAY/3 -> Terminator10/1
  BMS_RELAY/4 -> "BMS_RELAY "/1(In1)
  BMS_RELAY/5 -> Terminator2/1
  BMS_RELAY/2 -> Terminator43/1
  BMS_HCU_POWER/5 -> Terminator14/1
  BMS_HCU_POWER/2 -> Terminator12/1
  BMS_HCU_POWER/4 -> "BMS_HCU_POWER "/1(In1)
  BMS_HCU_POWER/3 -> Terminator13/1
  BMS_HCU_MAXT/3 -> Terminator25/1
  BMS_HCU_MAXT/2 -> Terminator24/1
  BMS_HCU_MAXT/5 -> Terminator26/1
  BMS_HCU_MAXT/1 -> BMS_HCU_MAXT1/Trigger
  BMS_HCU_MAXT/4 -> BMS_HCU_MAXT1/1(input)
  BMS_HCU_MAXV/4 -> "BMS_HCU_MAXV "/1(In1)
  BMS_HCU_MAXV/3 -> Terminator28/1
  BMS_HCU_MAXV/1 -> "BMS_HCU_MAXV "/Trigger
  BMS_HCU_MAXV/5 -> Terminator29/1
  BMS_HCU_MAXV/2 -> Terminator27/1
  BMS_HCU_POWER/1 -> "BMS_HCU_POWER "/Trigger
  "Motor_Current_Speed "/4 -> MOTOR_CURRENT_SPEED/1(input)
  "Motor_Current_Speed "/1 -> MOTOR_CURRENT_SPEED/Trigger
  "Motor_Current_Speed "/2 -> MeaModule/1
  "Motor_Current_Speed "/3 -> Terminator21/1
  "Motor_Current_Speed "/5 -> Terminator22/1
  BMS_HCU_MAXT1/1(HeatingCtl_Out) -> heatingctl/1
  BMS_HCU_MAXT1/2(CoolingCtl_Out) -> coolingctl/1
  BMS_HCU_MAXT1/3(MinTempNo_Out) -> mintempno/1
  BMS_HCU_MAXT1/4(MaxTempNo_Out) -> maxtempno/1
  BMS_HCU_MAXT1/5(MinTemp_Out) -> mintemp/1
  BMS_HCU_MAXT1/6(MaxTemp_Out) -> maxtemp/1
  "BMS_HCU_MAXV "/1(MaxCellVoltNo_Out) -> maxcellvoltno/1
  "BMS_HCU_MAXV "/3(MinCellVolt_Out) -> mincellvolt/1
  "BMS_HCU_MAXV "/4(MaxCellVolt_Out) -> maxcellvolt/1
  "BMS_HCU_MAXV "/2(MinCellVoltNo_Out) -> mincellvoltno/1
  "BMS_RELAY "/1(offChrRlyStr_Out) -> offChrRlyStr_Out/1
  "BMS_RELAY "/2(ChrReqCurr_Out) -> ChrReqCurr_Out/1
  "BMS_RELAY "/3(ChrReqVolt_Out) -> ChrReqVolt_Out/1
  "BMS_RELAY "/4(chrONCC_Out) -> chrONCC_Out/1
  "BMS_RELAY "/5(chrOFFCC2_Out) -> chrOFFCC2_Out/1
  "BMS_RELAY "/10(NegRlyStr_Out) -> NegRlyStr_Out/1
  "BMS_RELAY "/9(PreRlyStr_Out) -> PreRlyStr_Out/1
  "BMS_RELAY "/11(PosRlyStr_Out) -> PosRlyStr_Out/1
  "BMS_RELAY "/6(ChrCommunication_Out) -> ChrCommunication_Out/1
  "BMS_RELAY "/8(OnChrRlyStr_Out) -> OnChrRlyStr_Out/1
  "BMS_RELAY "/7(ChrState_Out) -> ChrState_Out/1
  "BMS_HCU_POWER "/3(MaxDisCurtLimit_Out) -> MaxDisCurtLimit_Out/1
  "BMS_HCU_POWER "/4(MaxChrCurtLimit_Out) -> MaxChrCurtLimit_Out/1
  "BMS_HCU_POWER "/1(MaxDisPowerLimit_Out) -> MaxDisPowerLimit_Out/1
  "BMS_HCU_POWER "/2(MaxChrPowerLimit_Out) -> MaxChrPowerLimit_Out/1
  MeaModule/1 -> Motor_Node/1
  MOTOR_CURRENT_SPEED/1(Motor_Currt_Speed_Out) -> Motor_Current_Speed/1
  "BMS_ALARM "/20(ALM_CELL_TBK_Out) -> ALM_CELL_TBK_Out/1
  "BMS_ALARM "/21(ALM_CELL_IBK_Out) -> ALM_CELL_IBK_Out/1
  "BMS_ALARM "/13(ALM_BATT_UC_Out) -> ALM_BATT_UC_Out/1
  "BMS_ALARM "/1(ALM_VCU_OFFLINE_Out) -> ALM_VCU_OFFLINE_Out/1
  "BMS_ALARM "/9(ALM_CHRG_OCS_Out) -> ALM_CHRG_OCS_Out/1
  "BMS_ALARM "/22(ALM_CELL_UT_Out) -> ALM_CELL_UT_Out/1
  "BMS_ALARM "/14(ALM_BATT_OC_Out) -> ALM_BATT_OC_Out/1
  "BMS_ALARM "/15(ALM_AUX_FAIL_Out) -> ALM_AUX_FAIL_Out/1
  "BMS_ALARM "/2(ALM_PRECHRG_FAIL_Out) -> ALM_PRECHRG_FAIL_Out/1
  "BMS_ALARM "/6(ALM_DSCH_OCT_Out) -> ALM_DSCH_OCT_Out/1
  "BMS_ALARM "/7(ALM_DSCH_OCS_Out) -> ALM_DSCH_OCS_Out/1
  "BMS_ALARM "/5(ALM_HALL_BREAK_Out) -> ALM_HALL_BREAK_Out/1
  "BMS_ALARM "/8(ALM_CHRG_OCT_Out) -> ALM_CHRG_OCT_Out/1
  "BMS_ALARM "/12(ALM_BMU_FAIL_Out) -> ALM_BMU_FAIL_Out/1
  "BMS_ALARM "/16(ALM_BATT_UV_Out) -> ALM_BATT_UV_Out/1
  "BMS_ALARM "/17(ALM_BATT_OV_Out) -> ALM_BATT_OV_Out/1
  "BMS_ALARM "/4(ALM_HVREL_FAIL_Out) -> ALM_HVREL_FAIL_Out/1
  "BMS_ALARM "/18(ALM_BATT_DT_Out) -> ALM_BATT_DT_Out/1
  "BMS_ALARM "/11(ALM_BSU_FAULT_Out) -> ALM_BSU_FAULT_Out/1
  "BMS_ALARM "/10(ALM_BSU_OFFLINE_Out) -> ALM_BSU_OFFLINE_Out/1
  "BMS_ALARM "/19(ALM_BATT_DV_Out) -> ALM_BATT_DV_Out/1
  "BMS_ALARM "/3(ALM_LEAK_OC_Out) -> ALM_LEAK_OC_Out/1
  "BMS_ALARM "/24(ALM_CELL_UV_Out) -> ALM_CELL_UV_Out/1
  "BMS_ALARM "/25(ALM_CELL_OV_Out) -> ALM_CELL_OV_Out/1
  "BMS_ALARM "/23(ALM_CELL_OT_Out) -> ALM_CELL_OT_Out/1

== system FSAC2021_V1_Running/VCU_CAN_Read/Subsystem ==
  function : TriggerPort  TriggerType=function-call
  BMS_HCU_INFO : ec55xxlib/RapidECU_U2/07CANCommucation/CANReceive  canmodule=B  canbuffer=54  canmessageid=2556444915  canmessagetype=Extended(29-bit ID)  datalength=8  sampletime=-1
  "BMS_HCU_INFO " : Subsystem
  MeaModule1 : ec55xxlib/RapidECU_U2/11Calibration/MeaModule  signal=bms_node
  Terminator16 : Terminator
  Terminator17 : Terminator
  BATLIFE : Outport
  BATALM : Outport  Port=2
  BATSTATE : Outport  Port=3
  BATSOH : Outport  Port=4
  BATSOC : Outport  Port=5
  BATCURRENT : Outport  Port=6
  BATVOLTAGLE : Outport  Port=7
  BMS_NODE : Outport  Port=8
  wires:
  "BMS_HCU_INFO "/7(BatVoltage_Out) -> BATVOLTAGLE/1
  "BMS_HCU_INFO "/6(BatCurrent_Out) -> BATCURRENT/1
  BMS_HCU_INFO/1 -> "BMS_HCU_INFO "/Trigger
  "BMS_HCU_INFO "/1(BatLife_Out) -> BATLIFE/1
  BMS_HCU_INFO/3 -> Terminator16/1
  "BMS_HCU_INFO "/5(BatSoc_Out) -> BATSOC/1
  "BMS_HCU_INFO "/2(BatAlmLv_Out) -> BATALM/1
  BMS_HCU_INFO/5 -> Terminator17/1
  "BMS_HCU_INFO "/3(BatState_Out) -> BATSTATE/1
  BMS_HCU_INFO/4 -> "BMS_HCU_INFO "/1(In1)
  BMS_HCU_INFO/2 -> MeaModule1/1
  "BMS_HCU_INFO "/4(BatSoh_Out) -> BATSOH/1
  MeaModule1/1 -> BMS_NODE/1

== system FSAC2021_V1_Running/VCU_CAN_Read/Subsystem1 ==
  function : TriggerPort  TriggerType=function-call
  HEARTBEAT : ec55xxlib/RapidECU_U2/07CANCommucation/CANReceive  canmodule=A  canbuffer=3  canmessageid=1793  canmessagetype=Standard(11-bit ID)  datalength=1  sampletime=-1
  "HEARTBEAT " : Subsystem
  MeaModule4 : ec55xxlib/RapidECU_U2/11Calibration/MeaModule  signal=motec_node
  Terminator : Terminator
  Terminator1 : Terminator
  Terminator2 : Terminator
  Motec_Node : Outport
  wires:
  HEARTBEAT/5 -> Terminator1/1
  HEARTBEAT/3 -> Terminator/1
  HEARTBEAT/4 -> "HEARTBEAT "/1(In1)
  HEARTBEAT/1 -> "HEARTBEAT "/Trigger
  HEARTBEAT/2 -> MeaModule4/1
  "HEARTBEAT "/1(Heartbeat_info_Out) -> Terminator2/1
  MeaModule4/1 -> Motec_Node/1

== system FSAC2021_V1_Running/VCU_CAN_Read/Subsystem2 ==
  function : TriggerPort  TriggerType=function-call
  MOTEC_STATUS : ec55xxlib/RapidECU_U2/07CANCommucation/CANReceive  canmodule=A  canbuffer=6  canmessageid=385  canmessagetype=Standard(11-bit ID)  datalength=2  sampletime=-1
  "MOTEC_STATUS " : Subsystem
  MeaModule5 : ec55xxlib/RapidECU_U2/11Calibration/MeaModule  signal=Steer_Status
  Terminator34 : Terminator
  Terminator35 : Terminator
  Str_Status : Outport
  Fault : Outport  Port=2
  operation_enable : Outport  Port=3
  quick_stop : Outport  Port=4
  ready_switch_on : Outport  Port=5
  switch_on_disable : Outport  Port=6
  switch_on : Outport  Port=7
  target_reached : Outport  Port=8
  voltagle_enable : Outport  Port=9
  warning_out : Outport  Port=10
  wires:
  "MOTEC_STATUS "/1(Fault_Out) -> Fault/1
  "MOTEC_STATUS "/2(Operation_Enabled_Out) -> operation_enable/1
  MOTEC_STATUS/5 -> Terminator35/1
  MOTEC_STATUS/3 -> Terminator34/1
  "MOTEC_STATUS "/3(Quick_Stop_Out) -> quick_stop/1
  "MOTEC_STATUS "/6(Swtiched_On_Out) -> switch_on/1
  "MOTEC_STATUS "/5(Switch_On_Disabled_Out) -> switch_on_disable/1
  MOTEC_STATUS/1 -> "MOTEC_STATUS "/Trigger
  "MOTEC_STATUS "/4(Ready_Switch_On_Out) -> ready_switch_on/1
  MOTEC_STATUS/4 -> "MOTEC_STATUS "/1(In1)
  MOTEC_STATUS/2 -> MeaModule5/1
  "MOTEC_STATUS "/8(Voltage_Enabled_Out) -> voltagle_enable/1
  "MOTEC_STATUS "/7(Target_Reached_Out) -> target_reached/1
  "MOTEC_STATUS "/9(Warning_Out) -> warning_out/1
  MeaModule5/1 -> Str_Status/1

== system FSAC2021_V1_Running/VCU_KL_Read/Read_VCU_AnaInput ==
  function : TriggerPort  TriggerType=function-call
  Gain : Gain  Gain=0.001  ParamDataTypeStr=single  OutDataTypeStr=single
  MeaModule : ec55xxlib/RapidECU_U2/11Calibration/MeaModule  signal=Read_Lft_Acc_Disp
  MeaModule1 : ec55xxlib/RapidECU_U2/11Calibration/MeaModule  signal=Read_Right_Acc_Disp1
  MeaModule2 : ec55xxlib/RapidECU_U2/11Calibration/MeaModule  signal=Read_Brk_Liquid_Prs
  MeaModule3 : ec55xxlib/RapidECU_U2/11Calibration/MeaModule  signal=Read_EBS_Gas_Prs1
  MeaModule4 : ec55xxlib/RapidECU_U2/11Calibration/MeaModule  signal=Read_EBS_Gas_Prs2
  MeaModule5 : ec55xxlib/RapidECU_U2/11Calibration/MeaModule  signal=Read_compare_OutVolt
  Read_Brk_Liquid_Prs : ec55xxlib/RapidECU_U2/02AnalogInput/AnalogInput  channel=54: I_AN15_5V  sampletime=-1
  Read_Compare : ec55xxlib/RapidECU_U2/02AnalogInput/AnalogInput  channel=73: I_AN19_5V  sampletime=-1
  Read_EBS_Gas_Prs1 : ec55xxlib/RapidECU_U2/02AnalogInput/AnalogInput  channel=56: I_AN17_5V  sampletime=-1
  Read_EBS_Gas_Prs2 : ec55xxlib/RapidECU_U2/02AnalogInput/AnalogInput  channel=71: I_AN18_5V  sampletime=-1
  Read_Lft_Acc_Disp : ec55xxlib/RapidECU_U2/02AnalogInput/AnalogInput  channel=53: I_AN14_5V  sampletime=-1
  Read_Right_Acc_Disp1 : ec55xxlib/RapidECU_U2/02AnalogInput/AnalogInput  channel=52: I_AN13_5V  sampletime=-1
  ACC_LEFT : Outport
  ACC_RIGHT : Outport  Port=2
  COMPARE_VOLTAGLE : Outport  Port=3
  BRK_LIQUID : Outport  Port=4
  EBS_GAS1 : Outport  Port=5
  EBS_GAS2 : Outport  Port=6
  wires:
  Read_EBS_Gas_Prs1/1 -> MeaModule3/1
  Read_Lft_Acc_Disp/1 -> MeaModule/1
  Read_Brk_Liquid_Prs/1 -> MeaModule2/1
  Read_Right_Acc_Disp1/1 -> MeaModule1/1
  Read_Compare/1 -> Gain/1
  Read_EBS_Gas_Prs2/1 -> MeaModule4/1
  Gain/1 -> MeaModule5/1
  MeaModule/1 -> ACC_LEFT/1
  MeaModule1/1 -> ACC_RIGHT/1
  MeaModule5/1 -> COMPARE_VOLTAGLE/1
  MeaModule2/1 -> BRK_LIQUID/1
  MeaModule3/1 -> EBS_GAS1/1
  MeaModule4/1 -> EBS_GAS2/1

== system FSAC2021_V1_Running/VCU_KL_Read/Read_VCU_DigInput ==
  function : TriggerPort  TriggerType=function-call
  ASMS_Read : ec55xxlib/RapidECU_U2/01SwitchInput/SwitchInput  channel=103: I_SW16_H  sampletime=-1
  Data Type Conversion{1..2,4,15..16,19,24..26} (9 alike) : DataTypeConversion  OutDataTypeStr=uint8
  EBS_Rel_Switch : ec55xxlib/RapidECU_U2/01SwitchInput/SwitchInput  channel=10: I_SW05_L  sampletime=-1
  HVMS_Read : ec55xxlib/RapidECU_U2/01SwitchInput/SwitchInput  channel=100: I_SW14_H  sampletime=-1
  HV_LIGHT : ec55xxlib/RapidECU_U2/01SwitchInput/SwitchInput  channel=112: I_SW19_H  sampletime=-1
  IMD_BENDER : ec55xxlib/RapidECU_U2/01SwitchInput/SwitchInput  channel=26: I_SW07_L  sampletime=-1
  LVMS_Read : ec55xxlib/RapidECU_U2/01SwitchInput/SwitchInput  channel=102: I_SW15_H  sampletime=-1
  MeaModule : ec55xxlib/RapidECU_U2/11Calibration/MeaModule  signal=LVMS_Read
  MeaModule1 : ec55xxlib/RapidECU_U2/11Calibration/MeaModule  signal=HVMS_Read
  MeaModule11 : ec55xxlib/RapidECU_U2/11Calibration/MeaModule  signal=On_IN_Switch
  MeaModule12 : ec55xxlib/RapidECU_U2/11Calibration/MeaModule  signal=START
  MeaModule13 : ec55xxlib/RapidECU_U2/11Calibration/MeaModule  signal=HV_LIGHT
  MeaModule14 : ec55xxlib/RapidECU_U2/11Calibration/MeaModule  signal=IMD_BENDER
  MeaModule2 : ec55xxlib/RapidECU_U2/11Calibration/MeaModule  signal=ASMS_Read
  MeaModule3 : ec55xxlib/RapidECU_U2/11Calibration/MeaModule  signal=On_Out_Switch
  MeaModule4 : ec55xxlib/RapidECU_U2/11Calibration/MeaModule  signal=EBS_Rel_Switch
  On_In_Switch : ec55xxlib/RapidECU_U2/01SwitchInput/SwitchInput  channel=104: I_SW17_H  sampletime=-1
  On_Out_Switch : ec55xxlib/RapidECU_U2/01SwitchInput/SwitchInput  channel=113: I_SW20_H  sampletime=-1
  START : ec55xxlib/RapidECU_U2/01SwitchInput/SwitchInput  channel=105: I_SW18_H  sampletime=-1
  LVMS : Outport
  HVMS : Outport  Port=2
  On_out_switch : Outport  Port=3
  Start : Outport  Port=4
  On_in_switch : Outport  Port=5
  HV_light : Outport  Port=6
  IMD_bender : Outport  Port=7
  EBS_Rel : Outport  Port=8
  ASMS : Outport  Port=9
  wires:
  On_In_Switch/1 -> MeaModule11/1
  HV_LIGHT/1 -> MeaModule13/1
  START/1 -> MeaModule12/1
  IMD_BENDER/1 -> MeaModule14/1
  LVMS_Read/1 -> MeaModule/1
  HVMS_Read/1 -> MeaModule1/1
  On_Out_Switch/1 -> MeaModule3/1
  EBS_Rel_Switch/1 -> MeaModule4/1
  MeaModule/1 -> Data Type Conversion19/1
  MeaModule1/1 -> Data Type Conversion1/1
  MeaModule3/1 -> Data Type Conversion15/1
  MeaModule4/1 -> Data Type Conversion16/1
  MeaModule11/1 -> Data Type Conversion24/1
  MeaModule12/1 -> Data Type Conversion25/1
  MeaModule13/1 -> Data Type Conversion26/1
  MeaModule14/1 -> Data Type Conversion2/1
  Data Type Conversion19/1 -> LVMS/1
  Data Type Conversion1/1 -> HVMS/1
  Data Type Conversion15/1 -> On_out_switch/1
  Data Type Conversion25/1 -> Start/1
  Data Type Conversion24/1 -> On_in_switch/1
  Data Type Conversion26/1 -> HV_light/1
  Data Type Conversion16/1 -> EBS_Rel/1
  Data Type Conversion2/1 -> IMD_bender/1
  Data Type Conversion4/1 -> ASMS/1
  ASMS_Read/1 -> MeaModule2/1
  MeaModule2/1 -> Data Type Conversion4/1

== system FSAC2021_V1_Running/VCU_KL_Read/Read_VCU_Freq(WheelSpeed) ==
  function : TriggerPort  TriggerType=function-call
  Read_FL_WhlSpd : ec55xxlib/RapidECU_U2/03FrequencyInput/FrequencyRead  Commented=on  channel=37: I_HALL1  sampletime=Ts
  Read_FR_WhlSpd : ec55xxlib/RapidECU_U2/03FrequencyInput/FrequencyRead  Commented=on  channel=38: I_HALL2  sampletime=Ts
  Read_RL_WhlSpd : ec55xxlib/RapidECU_U2/03FrequencyInput/FrequencyRead  channel=39: I_HALL3  sampletime=-1
  Read_RR_WhlSpd : ec55xxlib/RapidECU_U2/03FrequencyInput/FrequencyRead  channel=40: I_HALL4  sampletime=-1
  RL_WhlSpd_Hz : Outport
  RR_WhlSpd_Hz : Outport  Port=2
  wires:
  Read_RL_WhlSpd/1 -> RL_WhlSpd_Hz/1
  Read_RR_WhlSpd/1 -> RR_WhlSpd_Hz/1

== system FSAC2021_V1_Running/CAN_SEND/(BRK、STR、DRIVER)/BCU_MTR_MOVE_AB ==
  Brake_mtr_goalpos_in : Inport
  BCU_MTR_MOVE_AB_mux : Mux
  Brake_mtr_goalpos : Subsystem
  Conv{1..4} (4 alike) : DataTypeConversion
  output : Outport
  wires:
  BCU_MTR_MOVE_AB_mux/1 -> output/1
  Brake_mtr_goalpos/1(output1) -> Conv1/1
  Conv1/1 -> BCU_MTR_MOVE_AB_mux/1
  Brake_mtr_goalpos/2(output2) -> Conv2/1
  Conv2/1 -> BCU_MTR_MOVE_AB_mux/2
  Brake_mtr_goalpos/3(output3) -> Conv3/1
  Conv3/1 -> BCU_MTR_MOVE_AB_mux/3
  Brake_mtr_goalpos/4(output4) -> Conv4/1
  Conv4/1 -> BCU_MTR_MOVE_AB_mux/4
  Brake_mtr_goalpos_in/1 -> Brake_mtr_goalpos/1(Brake_mtr_goalpos)

== system FSAC2021_V1_Running/CAN_SEND/(BRK、STR、DRIVER)/BCU_STATUS_READ ==
  status_reg_num_in : Inport
  status_reg_addr_start_in : Inport  Port=2
  BCU_STATUS_READ_mux : Mux  Inputs=2
  Conv1 : DataTypeConversion
  Conv2 : DataTypeConversion
  status_reg_addr_start : Subsystem
  status_reg_num : Subsystem
  output : Outport
  wires:
  BCU_STATUS_READ_mux/1 -> output/1
  status_reg_addr_start/1(output1) -> Conv1/1
  Conv1/1 -> BCU_STATUS_READ_mux/1
  status_reg_num/1(output2) -> Conv2/1
  Conv2/1 -> BCU_STATUS_READ_mux/2
  status_reg_num_in/1 -> status_reg_num/1(status_reg_num)
  status_reg_addr_start_in/1 -> status_reg_addr_start/1(status_reg_addr_start)

== system FSAC2021_V1_Running/CAN_SEND/(BRK、STR、DRIVER)/MOTOR_SPEED_CONTROL ==
  Drive_Speed_Control_in : Inport
  Conv1 : DataTypeConversion
  Conv2 : DataTypeConversion
  Drive_Speed_Control : Subsystem
  MOTOR_SPEED_CONTROL_mux : Mux  Inputs=2
  output : Outport
  wires:
  MOTOR_SPEED_CONTROL_mux/1 -> output/1
  Drive_Speed_Control/1(output1) -> Conv1/1
  Conv1/1 -> MOTOR_SPEED_CONTROL_mux/1
  Drive_Speed_Control/2(output2) -> Conv2/1
  Conv2/1 -> MOTOR_SPEED_CONTROL_mux/2
  Drive_Speed_Control_in/1 -> Drive_Speed_Control/1(Drive_Speed_Control)

== system FSAC2021_V1_Running/CAN_SEND/(BRK、STR、DRIVER)/To_AMI ==
  vspd_in : Inport
  mtr_rpm_in : Inport  Port=2
  Battery_Volt_in : Inport  Port=3
  assi_status_in : Inport  Port=4
  Battery_Volt : Subsystem
  Conv{1..6} (6 alike) : DataTypeConversion
  To_AMI_mux : Mux  Inputs=8
  assi_status : Subsystem
  mtr_rpm : Subsystem
  vspd : Subsystem
  output : Outport
  wires:
  To_AMI_mux/1 -> output/1
  vspd/1(output1) -> Conv1/1
  Conv1/1 -> To_AMI_mux/1
  mtr_rpm/1(output2) -> Conv2/1
  Conv2/1 -> To_AMI_mux/2
  mtr_rpm/2(output3) -> Conv3/1
  Conv3/1 -> To_AMI_mux/3
  assi_status/1(output4) -> Conv4/1
  Conv4/1 -> To_AMI_mux/4
  Battery_Volt/1(output5) -> Conv5/1
  Conv5/1 -> To_AMI_mux/5
  Battery_Volt/2(output6) -> Conv6/1
  Conv6/1 -> To_AMI_mux/6
  vspd_in/1 -> vspd/1(vspd)
  mtr_rpm_in/1 -> mtr_rpm/1(mtr_rpm)
  Battery_Volt_in/1 -> Battery_Volt/1(Battery_Volt)
  assi_status_in/1 -> assi_status/1(assi_status)

== system FSAC2021_V1_Running/CAN_SEND/Subsystem/MOTOR_READ_SPEED ==
  Constant : Constant  Value=0  OutDataTypeStr=uint8
  MOTOR_READ_SPEED_mux : Mux  Inputs=8
  output : Outport
  wires:
  MOTOR_READ_SPEED_mux/1 -> output/1
  Constant/1 -> MOTOR_READ_SPEED_mux/1, MOTOR_READ_SPEED_mux/2, MOTOR_READ_SPEED_mux/3, MOTOR_READ_SPEED_mux/4, MOTOR_READ_SPEED_mux/8, MOTOR_READ_SPEED_mux/7, MOTOR_READ_SPEED_mux/6, MOTOR_READ_SPEED_mux/5

== system FSAC2021_V1_Running/CAN_SEND/Subsystem1/Brk_Mtr_Enbale ==
  BCU_MTR_ENABLE : Subsystem
  CANTransmit : ec55xxlib/RapidECU_U2/07CANCommucation/CANTransmit  canmodule=A  canbuffer=8  canmessageid=353  canmessagetype=Standard(11-bit ID)  datalength=8  sampletime=0.05
  MeaModule : ec55xxlib/RapidECU_U2/11Calibration/MeaModule  signal=BUC_Enable_Flag
  Terminator : Terminator
  wires:
  BCU_MTR_ENABLE/1(output) -> CANTransmit/1
  CANTransmit/1 -> MeaModule/1
  MeaModule/1 -> Terminator/1
